simulink model "two_link_random_ext_torque_dis"  (Simulink 8.7)
settings: Solver=FixedStepAuto  StartTime=0.0  StopTime=5  RelTol=1e-3
undefined symbols (not defined in the file or in its folder): DiscIntNeverNeededParam, dyn_return, external_cal_dis, external_cal_resi_dera_dis, P_cal_dis, resi_update_dis, two_link_gravity_position_control_dis, two_link_jacobian_dis
libraries: simulink x3
settings Model: Creator=Godric  LastModifiedBy=Godric
settings DataIOCC: LimitDataPoints=off  SaveFormat=Dataset
settings DebuggingCC: UnderspecifiedInitializationDetection=Simplified  MergeDetectMultiDrivingBlocksExec=error
settings HardwareCC: ProdBitPerPointer=64  ProdLargestAtomicFloat=Float  ProdIntDivRoundTo=Zero  ProdEndianess=LittleEndian  ProdWordSize=64  ProdHWDeviceType=Intel->x86-64 (Windows64)
settings ModelReferenceCC: PropagateSignalLabelsOutOfModel=on
settings ConfigComp: CovModelRefEnable=off

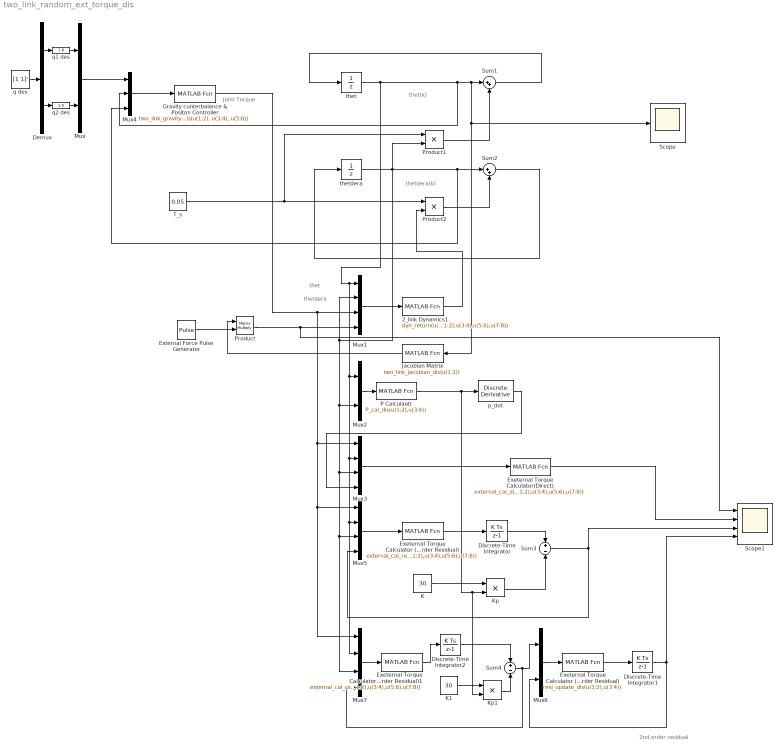
== system two_link_random_ext_torque_dis ==
  note: thetdera(k)
  note: thet(k)
  note: Joint Torque
  note: thetdera
  note: thet
  note: 2nd order residual
  2_link Dynamics1 : MATLABFcn  MATLABFcn=dyn_return(u(1:2),u(3:4),u(5:6),u(7:8))  OutputDimensions=[2,1]  Output1D=off
  Demux : Demux  Outputs=2
  Discrete-Time Integrator : DiscreteIntegrator  gainval=1  InitialConditionSetting=State (most efficient)  SampleTime=0.05  ICPrevOutput=DiscIntNeverNeededParam  ICPrevScaledInput=DiscIntNeverNeededParam
  Discrete-Time Integrator1 : DiscreteIntegrator  gainval=1  InitialConditionSetting=State (most efficient)  SampleTime=0.05  ICPrevOutput=DiscIntNeverNeededParam  ICPrevScaledInput=DiscIntNeverNeededParam
  Discrete-Time Integrator2 : DiscreteIntegrator  gainval=1  InitialConditionSetting=State (most efficient)  SampleTime=0.05  ICPrevOutput=DiscIntNeverNeededParam  ICPrevScaledInput=DiscIntNeverNeededParam
  Exeternal Torque Calculator (1-Order Residual) : MATLABFcn  MATLABFcn=external_cal_resi_dera_dis(u(1:2),u(3:4),u(5:6),u(7:8))  OutputDimensions=[2,1]  Output1D=off
  Exeternal Torque Calculator (1-Order Residual)1 : MATLABFcn  MATLABFcn=external_cal_resi_dera_dis(u(1:2),u(3:4),u(5:6),u(7:8))  OutputDimensions=[2,1]  Output1D=off
  Exeternal Torque Calculator (2-Order Residual) : MATLABFcn  MATLABFcn=resi_update_dis(u(1:2),u(3:4))  OutputDimensions=[2,1]  Output1D=off
  Exeternal Torque Calculator(Direct) : MATLABFcn  MATLABFcn=external_cal_dis(u(1:2),u(3:4),u(5:6),u(7:8))  OutputDimensions=[2,1]  Output1D=off
  External Force Pulse Generator : DiscretePulseGenerator  PulseType=Time based  Amplitude=[12 14]'  Period=20  PulseWidth=0.25  PhaseDelay=4
  Gravity cunterbalance & Positon Controller : MATLABFcn  MATLABFcn=two_link_gravity_position_control_dis(u(1:2), u(3:4), u(5:6))  OutputDimensions=[2,1]  Output1D=off
  Jacobian Matrix : MATLABFcn  MATLABFcn=two_link_jacobian_dis(u(1:2))  OutputDimensions=[2,2]  OutputSignalType=real  Output1D=off
  K : Constant  Value=30
  K1 : Constant  Value=30
  Kp : Product
  Kp1 : Product
  Mux : Mux  Inputs=2
  Mux{1,3,5,7} (4 alike) : Mux
  Mux2 : Mux  Inputs=2
  Mux4 : Mux  Inputs=3
  Mux6 : Mux  Inputs=2
  P Calculaotr : MATLABFcn  MATLABFcn=P_cal_dis(u(1:2),u(3:4))  OutputDimensions=[2,1]  Output1D=off
  Product : Product  Multiplication=Matrix(*)
  Product1 : Product
  Product2 : Product
  Scope : Scope
  Scope1 : Scope  NumInputPorts=4
  Sum1 : Sum  Inputs=|++
  Sum2 : Sum  Inputs=|++
  Sum3 : Sum  Inputs=+-
  Sum4 : Sum  Inputs=+-
  T_s : Constant  Value=0.05
  p_dot : simulink/Discrete/Discrete Derivative  gainval=1.0  ICPrevScaledInput=0.0  OutMin=[]  OutMax=[]  OutDataType=fixdt(1, 16)  OutScaling=2^-10  DoSatur=off
  q des : Constant  Value=[1 1]'
  q1 des : simulink/Math Operations/Slider Gain  low=-2  gain=1.8  high=2
  q2 des : simulink/Math Operations/Slider Gain  low=-2  gain=1.5  high=2
  thet : UnitDelay  InitialCondition=[0 0]'  SampleTime=0.05
  thetdera : UnitDelay  InitialCondition=[0 0]'  SampleTime=0.05
  wires:
  Demux/1 -> q1 des/1
  Demux/2 -> q2 des/1
  q2 des/1 -> Mux/2
  q1 des/1 -> Mux/1
  q des/1 -> Demux/1
  Mux/1 -> Mux4/1
  Mux4/1 -> Gravity cunterbalance & Positon Controller/1
  Gravity cunterbalance & Positon Controller/1 -> Mux7/1, Mux5/1, Mux3/1, Mux1/3
  thet/1 -> Mux7/2, Mux5/2, Mux3/2, Mux2/1, Mux1/1, Scope/1, Jacobian Matrix/1, Sum1/1, Mux4/2
  Product1/1 -> Sum1/2
  T_s/1 -> Product1/1, Product2/1
  thetdera/1 -> Mux1/2, Mux7/3, Mux5/3, Mux3/3, Mux2/2, Mux4/3, Sum2/1, Product1/2
  Sum1/1 -> thet/1
  Product2/1 -> Sum2/2
  Sum2/1 -> thetdera/1
  Mux1/1 -> 2_link Dynamics1/1
  2_link Dynamics1/1 -> Product2/2
  Product/1 -> Scope1/1, Mux1/4
  Jacobian Matrix/1 -> Product/1
  External Force Pulse Generator/1 -> Product/2
  Mux2/1 -> P Calculaotr/1
  P Calculaotr/1 -> p_dot/1, Kp1/2, Kp/2
  Mux3/1 -> Exeternal Torque Calculator(Direct)/1
  p_dot/1 -> Mux3/4
  Mux5/1 -> Exeternal Torque Calculator (1-Order Residual)/1
  K/1 -> Kp/1
  Kp/1 -> Sum3/2
  Sum3/1 -> Scope1/3, Mux5/4
  Exeternal Torque Calculator (1-Order Residual)/1 -> Discrete-Time Integrator/1
  Discrete-Time Integrator/1 -> Sum3/1
  Mux6/1 -> Exeternal Torque Calculator (2-Order Residual)/1
  Exeternal Torque Calculator (2-Order Residual)/1 -> Discrete-Time Integrator1/1
  K1/1 -> Kp1/1
  Mux7/1 -> Exeternal Torque Calculator (1-Order Residual)1/1
  Exeternal Torque Calculator (1-Order Residual)1/1 -> Discrete-Time Integrator2/1
  Kp1/1 -> Sum4/2
  Sum4/1 -> Mux7/4, Mux6/1
  Discrete-Time Integrator1/1 -> Mux6/2, Scope1/4
  Discrete-Time Integrator2/1 -> Sum4/1
  Exeternal Torque Calculator(Direct)/1 -> Scope1/2
